simulink model "HW8"  (R2016a)
settings: Solver=VariableStepAuto  StartTime=0.0  StopTime=10  RelTol=1e-3
settings Model: Creator=古乔  LastModifiedBy=古乔

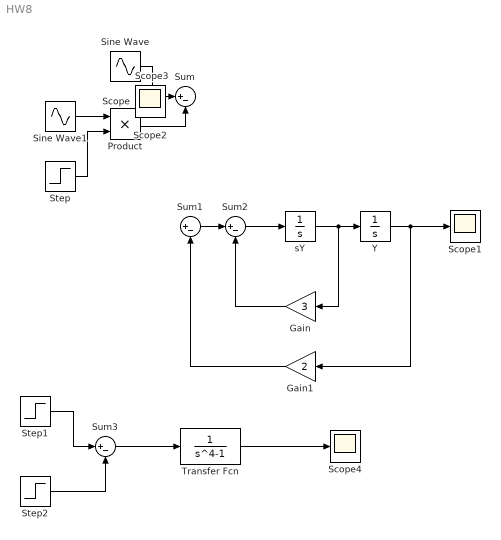
== system HW8 ==
  Gain : Gain  Gain=3
  Gain1 : Gain  Gain=2
  Product : Product
  Scope{,1..4} (5 alike) : Scope
  Sine Wave : Sin  SampleTime=0
  Sine Wave1 : Sin  Amplitude=-1  Phase=-pi  SampleTime=0
  Step : Step  Time=pi  SampleTime=0
  Step1 : Step  SampleTime=0
  Step2 : Step  Time=3  SampleTime=0
  Sum{,1..3} (4 alike) : Sum  Inputs=|+-
  Transfer Fcn : TransferFcn  Denominator=[1 0 0 0 -1]
  Y : Integrator  InitialCondition=1
  sY : Integrator
  wires:
  Sine Wave/1 -> Sum/1
  Product/1 -> Sum/2
  sY/1 -> Gain/1, Y/1
  Y/1 -> Scope1/1, Gain1/1
  Sum2/1 -> sY/1
  Sum1/1 -> Sum2/1
  Gain/1 -> Sum2/2
  Gain1/1 -> Sum1/2
  Sine Wave1/1 -> Product/1
  Step/1 -> Product/2
  Step1/1 -> Sum3/1
  Step2/1 -> Sum3/2
  Sum3/1 -> Transfer Fcn/1
  Transfer Fcn/1 -> Scope4/1
